simulink library "dc_motor_lib"  (R2016b)
settings: Solver=VariableStepAuto  StartTime=0.0  StopTime=10.0  RelTol=1e-3
undefined symbols (not defined in the file): sim_params
settings Model: Creator=Taylor  LastModifiedBy=Taylor

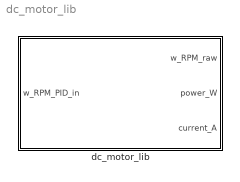
== system dc_motor_lib ==
  dc_motor_lib : Subsystem

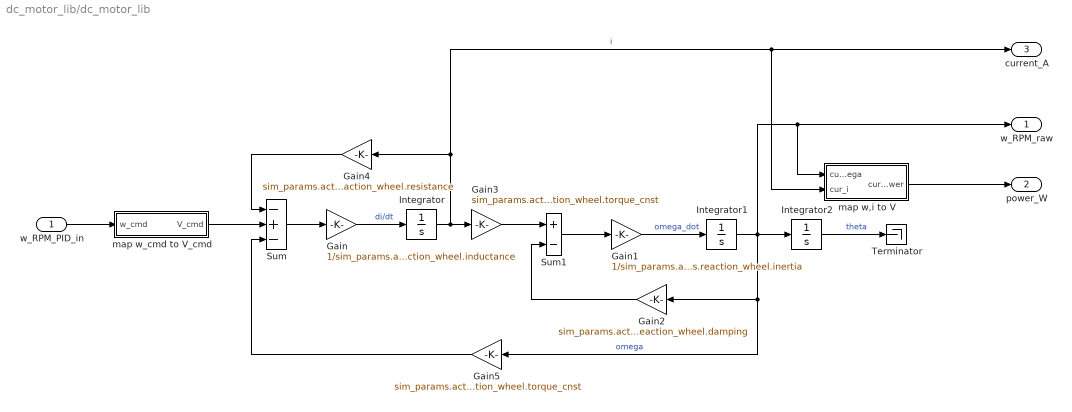
== system dc_motor_lib/dc_motor_lib ==
  w_RPM_PID_in : Inport
  Gain : Gain  Gain=1/sim_params.actuators.reaction_wheel.inductance
  Gain1 : Gain  Gain=1/sim_params.actuators.reaction_wheel.inertia
  Gain2 : Gain  Gain=sim_params.actuators.reaction_wheel.damping
  Gain3 : Gain  Gain=sim_params.actuators.reaction_wheel.torque_cnst
  Gain4 : Gain  Gain=sim_params.actuators.reaction_wheel.resistance
  Gain5 : Gain  Gain=sim_params.actuators.reaction_wheel.torque_cnst
  Integrator : Integrator  InitialCondition=sim_params.actuators.reaction_wheel.ic.current
  Integrator1 : Integrator  InitialCondition=sim_params.actuators.reaction_wheel.ic.omega
  Integrator2 : Integrator  InitialCondition=sim_params.actuators.reaction_wheel.ic.theta
  Sum : Sum  Inputs=-+-
  Sum1 : Sum  Inputs=+-
  Terminator : Terminator
  map w,i to V : Subsystem
  map w_cmd to V_cmd : Subsystem
  w_RPM_raw : Outport
  power_W : Outport  Port=2
  current_A : Outport  Port=3
  wires:
  Gain4/1 -> Sum/1
  Sum1/1 -> Gain1/1
  Gain1/1 -> Integrator1/1  "omega_dot"
  Integrator2/1 -> Terminator/1  "theta"
  Gain/1 -> Integrator/1  "di/dt"
  Gain2/1 -> Sum1/2
  Gain5/1 -> Sum/3
  Gain3/1 -> Sum1/1
  map w_cmd to V_cmd/1(V_cmd) -> Sum/2
  map w,i to V/1(cur_power) -> power_W/1
  Integrator1/1 -> w_RPM_raw/1, map w,i to V/1(cur_omega), Gain5/1, Gain2/1, Integrator2/1  "omega"
  Sum/1 -> Gain/1
  w_RPM_PID_in/1 -> map w_cmd to V_cmd/1(w_cmd)
  Integrator/1 -> current_A/1, map w,i to V/2(cur_i), Gain4/1, Gain3/1  "i"

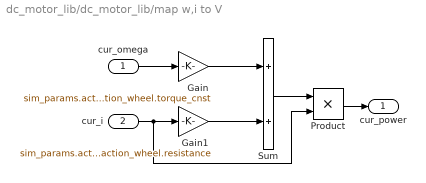
== system dc_motor_lib/dc_motor_lib/map w,i to V ==
  cur_omega : Inport
  cur_i : Inport  Port=2
  Gain : Gain  Gain=sim_params.actuators.reaction_wheel.torque_cnst
  Gain1 : Gain  Gain=sim_params.actuators.reaction_wheel.resistance
  Product : Product
  Sum : Sum
  cur_power : Outport
  wires:
  cur_omega/1 -> Gain/1
  Gain/1 -> Sum/1
  Gain1/1 -> Sum/2
  Sum/1 -> Product/1
  cur_i/1 -> Product/2, Gain1/1
  Product/1 -> cur_power/1

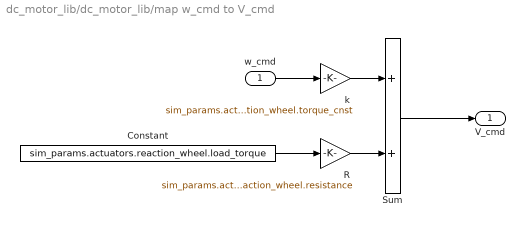
== system dc_motor_lib/dc_motor_lib/map w_cmd to V_cmd ==
  w_cmd : Inport
  Constant : Constant  Value=sim_params.actuators.reaction_wheel.load_torque
  "R " : Gain  Gain=sim_params.actuators.reaction_wheel.resistance
  Sum : Sum
  k : Gain  Gain=sim_params.actuators.reaction_wheel.torque_cnst
  V_cmd : Outport
  wires:
  w_cmd/1 -> k/1
  k/1 -> Sum/1
  Constant/1 -> "R "/1
  "R "/1 -> Sum/2
  Sum/1 -> V_cmd/1
